simulink model "Prac3Simu (1)"  (R2024b)
settings: Solver=VariableStepAuto  StartTime=0.0  StopTime=10.0  MaxStep=0.01  RelTol=1e-3
InitFcn:
  | m1 = 290;
  | b1 = 1000;
  | m2 = 59;
  | k1 = 16182;
  | f = 0;
  | k2 = 19000;

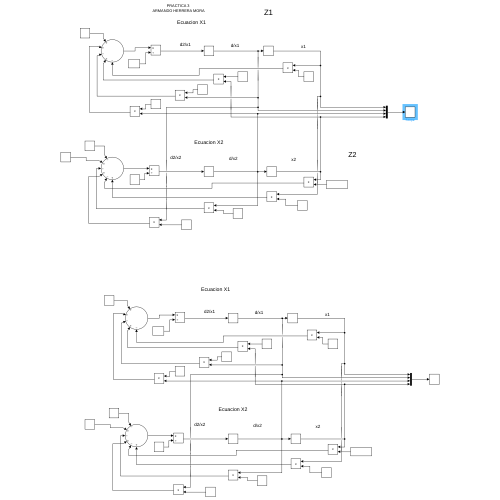
[thumbnail: Simulink's stored preview of the top-level diagram]
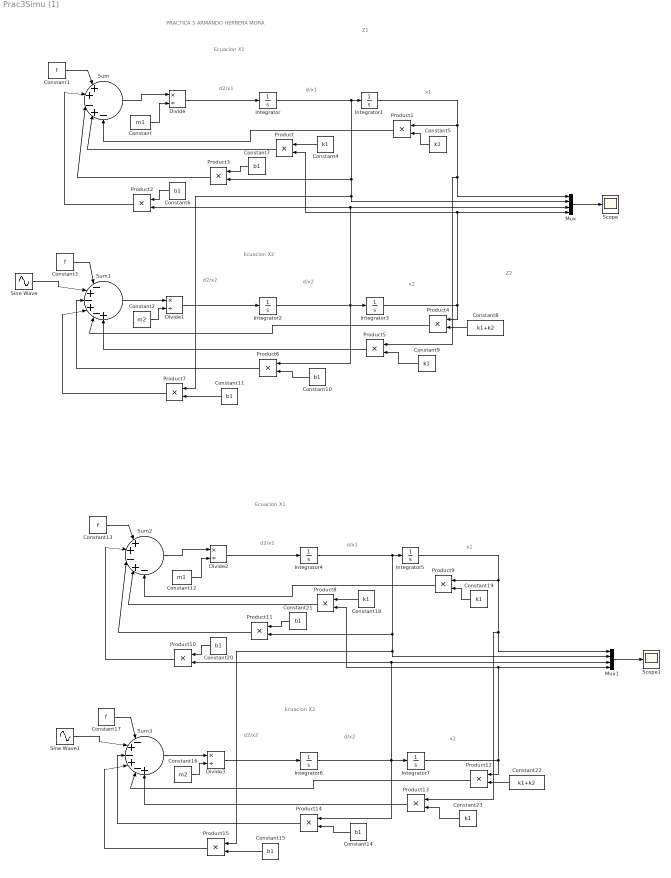
== system Prac3Simu (1) ==
  note: Z2
  note: Z1
  note: Ecuacion X1
  note: PRACTICA 3
      | ARMANDO HERRERA MORA
  note: d2/x1
  note: x1
  note: d/x1
  note: d2/x2
  note: x2
  note: Ecuacion X2
  note: d/x2
  note: Ecuacion X2
  note: x2
  note: d2/x2
  note: x1
  note: d2/x1
  note: d/x2
  note: Ecuacion X1
  note: d/x1
  Constant : Constant  Value=m1
  Constant{1,3,13,17} (4 alike) : Constant  Value=f
  Constant{6..7,10..11,14..15,20..21} (8 alike) : Constant  Value=b1
  Constant12 : Constant  Value=m1
  Constant16 : Constant  Value=m2
  Constant{4..5,9,18..19,23} (6 alike) : Constant  Value=k1
  Constant2 : Constant  Value=m2
  Constant22 : Constant  Value=k1+k2
  Constant8 : Constant  Value=k1+k2
  Divide{,1..3} (4 alike) : Product  Inputs=*/
  Integrator{,1..7} (8 alike) : Integrator
  Mux : Mux
  Mux1 : Mux
  Product{,1..15} (16 alike) : Product
  Scope : Scope
  Scope1 : Scope
  Sine Wave : Sin  Amplitude=0.05  Frequency=0.5*pi  SampleTime=0
  Sine Wave1 : Sin  Amplitude=0.05  Frequency=20*pi  SampleTime=0
  Sum : Sum  Inputs=|++-+-
  Sum1 : Sum  Inputs=|-+-+-+
  Sum2 : Sum  Inputs=|++-+-
  Sum3 : Sum  Inputs=|-+-+-+
  wires:
  Sum/1 -> Divide/1
  Constant/1 -> Divide/2
  Constant1/1 -> Sum/1
  Mux/1 -> Scope/1
  Divide/1 -> Integrator/1
  Integrator/1 -> Product7/1, Mux/2, Product3/2, Integrator1/1
  Integrator1/1 -> Product1/1, Product5/1, Mux/1
  Sum1/1 -> Divide1/1
  Constant2/1 -> Divide1/2
  Divide1/1 -> Integrator2/1
  Integrator3/1 -> Product4/1, Mux/4, Product/2
  Integrator2/1 -> Product6/1, Product2/2, Mux/3, Integrator3/1
  Constant3/1 -> Sum1/1
  Constant4/1 -> Product/1
  Constant5/1 -> Product1/2
  Product1/1 -> Sum/5
  Constant6/1 -> Product2/1
  Product/1 -> Sum/4
  Product2/1 -> Sum/2
  Constant7/1 -> Product3/1
  Product3/1 -> Sum/3
  Constant8/1 -> Product4/2
  Product4/1 -> Sum1/5
  Constant9/1 -> Product5/2
  Product5/1 -> Sum1/6
  Constant10/1 -> Product6/2
  Product6/1 -> Sum1/3
  Constant11/1 -> Product7/2
  Product7/1 -> Sum1/4
  Sine Wave/1 -> Sum1/2
  Mux1/1 -> Scope1/1
  Constant18/1 -> Product8/1
  Integrator6/1 -> Product14/1, Product10/2, Mux1/3, Integrator7/1
  Integrator5/1 -> Product9/1, Product13/1, Mux1/1
  Sine Wave1/1 -> Sum3/2
  Constant17/1 -> Sum3/1
  Product11/1 -> Sum2/3
  Product12/1 -> Sum3/5
  Integrator7/1 -> Product12/1, Mux1/4, Product8/2
  Constant20/1 -> Product10/1
  Constant16/1 -> Divide3/2
  Divide2/1 -> Integrator4/1
  Product8/1 -> Sum2/4
  Product15/1 -> Sum3/4
  Constant21/1 -> Product11/1
  Constant15/1 -> Product15/2
  Constant12/1 -> Divide2/2
  Constant13/1 -> Sum2/1
  Constant19/1 -> Product9/2
  Constant22/1 -> Product12/2
  Product9/1 -> Sum2/5
  Constant14/1 -> Product14/2
  Integrator4/1 -> Product15/1, Mux1/2, Product11/2, Integrator5/1
  Product14/1 -> Sum3/3
  Divide3/1 -> Integrator6/1
  Constant23/1 -> Product13/2
  Product10/1 -> Sum2/2
  Product13/1 -> Sum3/6
  Sum3/1 -> Divide3/1
  Sum2/1 -> Divide2/1
